simulink model "pvs_series_resonant_converter"  (R2021a)
settings: Solver=VariableStepAuto  StartTime=0.0  StopTime=0.005  RelTol=1e-3
libraries: spsDiodeLib x4, spsSeriesRLCBranchLib x4, spsCurrentMeasurementLib x2, spsMosfetLib x2, spsLinearTransformerLib x1, spsPVArrayLib x1, spsVoltageMeasurementLib x1, spspowerguiLib x1
settings Model: Creator=ADMIN  LastModifiedBy=ADMIN

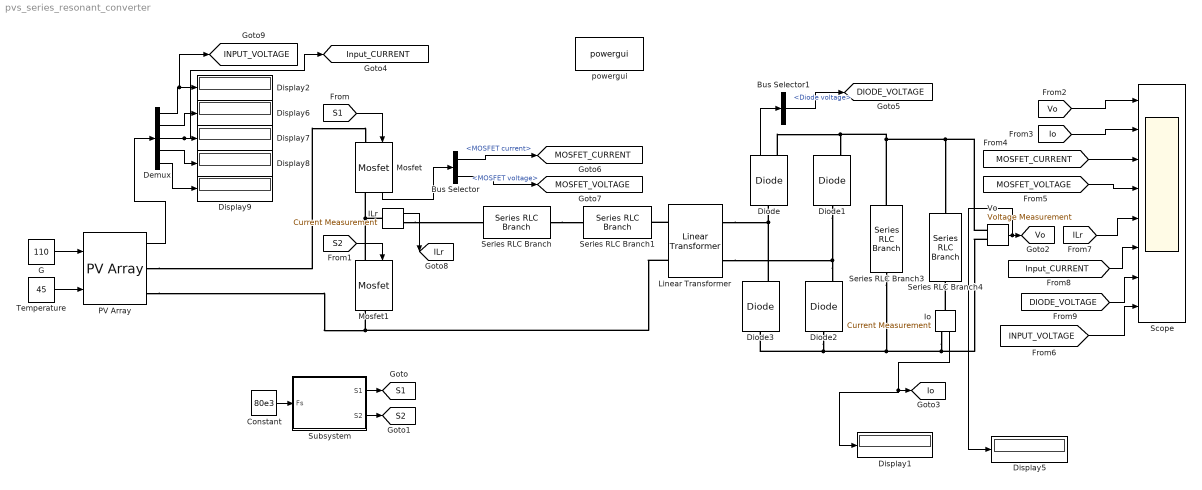
== system pvs_series_resonant_converter ==
  Bus Selector : BusSelector  OutputSignals=MOSFET current,MOSFET voltage
  Bus Selector1 : BusSelector  OutputSignals=Diode voltage
  Constant : Constant  Value=80e3
  Demux : Demux  Outputs=5
  Diode{,1..3} (4 alike) : spsDiodeLib/Diode  Ron=0.001  Lon=0  Vf=0.8  IC=0  UseSnubber=0  Rs=500  Cs=250e-9  Measurements=on
  Display{1..2,5..9} (7 alike) : Display
  G : Constant  Value=110
  ILr : spsCurrentMeasurementLib/Current Measurement  PhasorSimulation=off  OutputType=Complex  PSBequivalent=0
  Io : spsCurrentMeasurementLib/Current Measurement  PhasorSimulation=off  OutputType=Complex  PSBequivalent=0
  Linear Transformer : spsLinearTransformerLib/Linear Transformer  UNITS=SI  NominalPower=[ 200 200e3 ]  winding1=[3.39 0 0]  winding2=[1 0 0]  ThreeWindings=off  winding3=[3.15e+05 0.7938 0.084225]  RmLm=[100 0]  Measurements=None  DataType=on
  Mosfet : spsMosfetLib/Mosfet  Ron=0.1  Lon=0  Rd=0.01  Vfd=0  IC=0  Rs=1e5  Cs=inf  Measurements=on
  Mosfet1 : spsMosfetLib/Mosfet  Ron=0.1  Lon=0  Rd=0.01  Vfd=0  IC=0  Rs=1e5  Cs=inf  Measurements=on
  PV Array : spsPVArrayLib/PV Array  Npar=1  Nser=1  PlotType=array @ 1000 W/m2 & specified temperatures  S_vec="[ 1000  500  100 ]"  Temp_C_vec="[ 45 25  ]"  ModuleName=Hanwha SolarOne (Qidong) SF160-24-M150  PlotWhenSelected=off  Pm=149.988  Ncell=72  Voc=43.4  Isc=4.88  Vm=34.8  Im=4.31  beta_Voc_pc=-0.328  alpha_Isc_pc=0.033996  beta_Voc=-0.14235  alpha_Isc=0.001659  IL=4.9254  I0=4.7771e-11  nI=0.92869  Rsh=95.9331  Rs=0.79087  RobustModel=off  RobustCellTemperature=313.3991  BAL=off  Tc=1e-6  Tfilter=5e-5
  Scope : Scope  NumInputPorts=8
  Series RLC Branch : spsSeriesRLCBranchLib/Series RLC Branch  LConnTagsString=__new0  RConnTagsString=__new0  BranchType=L  Resistance=1  Inductance=15e-6  SetiL0=off  InitialCurrent=0  Capacitance=1e-6  Setx0=off  InitialVoltage=0  Measurements=None
  Series RLC Branch1 : spsSeriesRLCBranchLib/Series RLC Branch  LConnTagsString=__new0  RConnTagsString=__new0  BranchType=C  Resistance=1  Inductance=1e-3  SetiL0=off  InitialCurrent=0  Capacitance=29e-9  Setx0=off  InitialVoltage=0  Measurements=None
  Series RLC Branch3 : spsSeriesRLCBranchLib/Series RLC Branch  LConnTagsString=__new0  RConnTagsString=__new0  BranchType=C  Resistance=1  Inductance=1e-3  SetiL0=off  InitialCurrent=0  Capacitance=1e-6  Setx0=off  InitialVoltage=0  Measurements=None
  Series RLC Branch4 : spsSeriesRLCBranchLib/Series RLC Branch  LConnTagsString=__new0  RConnTagsString=__new0  BranchType=R  Resistance=300  Inductance=1e-3  SetiL0=off  InitialCurrent=0  Capacitance=1e-6  Setx0=off  InitialVoltage=0  Measurements=None
  Subsystem : Subsystem
  Temperature : Constant  Value=45
  Vo : spsVoltageMeasurementLib/Voltage Measurement  PhasorSimulation=off  OutputType=Complex  PSBequivalent=0
  powergui : spspowerguiLib/powergui  Priority=1  SimulationMode=Continuous  SampleTime=50e-6  frequency=60  Iterations=50  frequencyindice=0  Pbase=100e6  ErrMax=1e-4  UnitsV=kV  UnitsW=MW  buscounter=0  FunctionMessages=off  echomessages=off  EnableUseOfTLC=off  CurrentSourceSwitches=off  DisableSnubberDevices=off  DisableRonSwitches=off  DisableVfSwitches=off  DisplayEquations=off  AutomaticDiscreteSolvers=off  SolverType=Tustin/Backward Euler (TBE)  Interpol=off  ExternalGateDelay=off  methode=off  Ts=100  x0status=blocks  SPID=on  SwTol=0  HookPort=off  NonlinearTolerance=0  nMaxIteration=15  ContinueOnMaxIteration=off  RestoreLinks=warning  ResistiveCurrentMeasurement=off  Frange=[0:2:500]  Ylog=off  Xlog=on  ShowGrid=off  save=off  variable=ZData  structure=0  ZoomFFT=off  StartTime=0.0  cycles=1  DisplayStyle=1  fundamental=60  FreqAxis=off  MaxFrequency=1000  frequencyindicesteady=1  RmsSteady=1  display=off
  tag scope: DIODE_VOLTAGE=global, ILr=global, INPUT_VOLTAGE=global, Input_CURRENT=global, Io=global, MOSFET_CURRENT=global, MOSFET_VOLTAGE=global, S1=global, S2=global, Vo=global
  wires:
  Demux/1 -> [INPUT_VOLTAGE], Display2/1
  Io/1 -> Display1/1, [Io]
  ILr/1 -> [ILr]
  Demux/5 -> Display9/1
  Demux/2 -> Display6/1
  [Io] -> Scope/2
  [S2] -> Mosfet1/1
  [MOSFET_CURRENT] -> Scope/3
  Constant/1 -> Subsystem/1(" Fs")
  [S1] -> Mosfet/1
  Subsystem/2(S2) -> [S2]
  PV Array/1 -> Demux/1
  [Vo] -> Scope/1
  Bus Selector/2 -> [MOSFET_VOLTAGE]  "<MOSFET voltage>"
  [ILr] -> Scope/5
  Diode/1 -> Bus Selector1/1
  Temperature/1 -> PV Array/2
  Demux/4 -> Display8/1
  Mosfet/1 -> Bus Selector/1
  [MOSFET_VOLTAGE] -> Scope/4
  G/1 -> PV Array/1
  Vo/1 -> Display5/1, [Vo]
  Subsystem/1(S1) -> [S1]
  [INPUT_VOLTAGE] -> Scope/8
  Bus Selector1/1 -> [DIODE_VOLTAGE]  "<Diode voltage>"
  Demux/3 -> [Input_CURRENT], Display7/1
  [DIODE_VOLTAGE] -> Scope/7
  [Input_CURRENT] -> Scope/6
  Bus Selector/1 -> [MOSFET_CURRENT]  "<MOSFET current>"
  connections:
  Mosfet1/RConn1 -- Linear Transformer/LConn2 -- PV Array/RConn2
  Mosfet/RConn1 -- Mosfet1/LConn1 -- ILr/LConn1
  Diode3/LConn1 -- Diode2/LConn1 -- Vo/LConn2 -- Io/RConn1 -- Series RLC Branch3/RConn1
  Series RLC Branch3/LConn1 -- Vo/LConn1 -- Series RLC Branch4/LConn1 -- Diode/RConn1 -- Diode1/RConn1
  Diode/LConn1 -- Diode3/RConn1 -- Linear Transformer/RConn1
  Diode2/RConn1 -- Diode1/LConn1 -- Linear Transformer/RConn2
  Series RLC Branch/RConn1 -- Series RLC Branch1/LConn1
  Io/LConn1 -- Series RLC Branch4/RConn1
  PV Array/RConn1 -- Mosfet/LConn1
  Linear Transformer/LConn1 -- Series RLC Branch1/RConn1
  ILr/RConn1 -- Series RLC Branch/LConn1

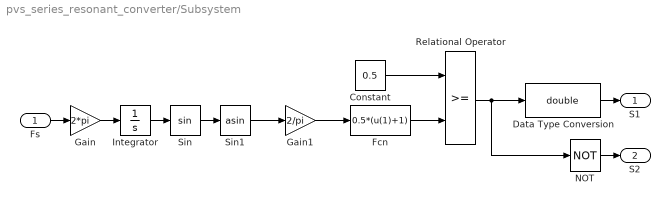
== system pvs_series_resonant_converter/Subsystem ==
  " Fs" : Inport
  Constant : Constant  Value=0.5
  Data Type Conversion : DataTypeConversion  OutDataTypeStr=double
  Fcn : Fcn  Expr=0.5*(u(1)+1)
  Gain : Gain  Gain=2*pi
  Gain1 : Gain  Gain=2/pi
  Integrator : Integrator
  NOT : Logic  Operator=NOT  IconShape=distinctive  AllPortsSameDT=off  OutDataTypeStr=boolean
  Relational Operator : RelationalOperator  OutDataTypeStr=boolean  RndMeth=Simplest
  Sin : Trigonometry
  Sin1 : Trigonometry  Operator=asin
  S1 : Outport  VectorParamsAs1DForOutWhenUnconnected=off
  S2 : Outport  Port=2  VectorParamsAs1DForOutWhenUnconnected=off
  wires:
  Integrator/1 -> Sin/1
  Constant/1 -> Relational Operator/1
  Sin1/1 -> Gain1/1
  Sin/1 -> Sin1/1
  Relational Operator/1 -> NOT/1, Data Type Conversion/1
  Gain/1 -> Integrator/1
  Gain1/1 -> Fcn/1
  Fcn/1 -> Relational Operator/2
  NOT/1 -> S2/1
  " Fs"/1 -> Gain/1
  Data Type Conversion/1 -> S1/1
